simulink model "Q_robot_control_walk_SPT5425"  (R2018b)
settings: Solver=FixedStepAuto  StartTime=0.0  StopTime=10  FixedStep=0.01  RelTol=1e-3
libraries: simulink x3
settings Model: Creator=lsl  LastModifiedBy=lsl

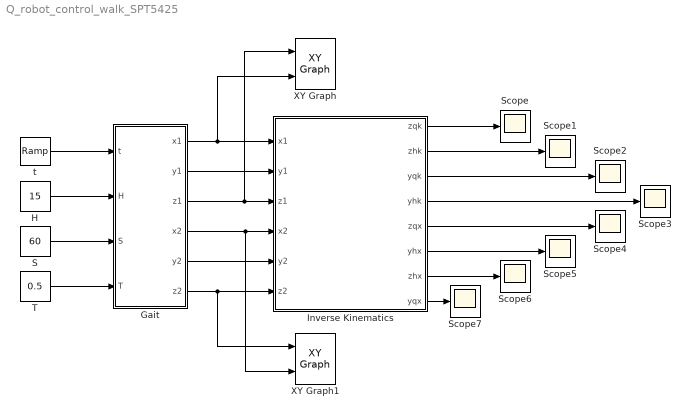
== system Q_robot_control_walk_SPT5425 ==
  Gait : MATLAB Function  TreatAsAtomicUnit=on
  H : Constant  Value=15
  Inverse Kinematics : MATLAB Function  TreatAsAtomicUnit=on
  S : Constant  Value=60
  Scope{,1..7} (8 alike) : Scope
  T : Constant  Value=0.5
  XY Graph : simulink/Sinks/XY Graph  xmin=-100  xmax=100  ymin=-100  ymax=100  st=-1
  XY Graph1 : simulink/Sinks/XY Graph  xmin=-100  xmax=100  ymin=-100  ymax=100  st=-1
  t : simulink/Sources/Ramp  slope=1  start=0  InitialOutput=0
  wires:
  t/1 -> Gait/1(t)
  T/1 -> Gait/4(T)
  Gait/5(y2) -> Inverse Kinematics/5(y2)
  Gait/3(z1) -> XY Graph/1, Inverse Kinematics/3(z1)
  Gait/2(y1) -> Inverse Kinematics/2(y1)
  Gait/1(x1) -> XY Graph/2, Inverse Kinematics/1(x1)
  Inverse Kinematics/6(yhx) -> Scope5/1
  Inverse Kinematics/1(zqk) -> Scope/1
  Inverse Kinematics/7(zhx) -> Scope6/1
  Gait/4(x2) -> XY Graph1/2, Inverse Kinematics/4(x2)
  Gait/6(z2) -> XY Graph1/1, Inverse Kinematics/6(z2)
  Inverse Kinematics/2(zhk) -> Scope1/1
  Inverse Kinematics/3(yqk) -> Scope2/1
  Inverse Kinematics/4(yhk) -> Scope3/1
  Inverse Kinematics/5(zqx) -> Scope4/1
  Inverse Kinematics/8(yqx) -> Scope7/1
  S/1 -> Gait/3(S)
  H/1 -> Gait/2(H)

== matlab function Q_robot_control_walk_SPT5425/Gait ==
  data: t input; H input; x1 output; S input; T input; y1 output; z1 output; x2 output; y2 output; z2 output
function [x1,y1,z1,x2,y2,z2] = Gait_SPT(t,H,S,T)
%x1,y1,z1 摆动相
%x2,y2,z2 支撑相
SwayStatus_Xst=170;
SwayStatus_Yst=43.9;
SwayStatus_Zst=-0.5*S;

SupportingStatus_Xst=170;
SupportingStatus_Yst=43.9;
SupportingStatus_Zst=0.5*S;

if(t>T)
    c=mod(t,T);
else 
    c=t;
end
temp=(t-c)/T;
if(mod(temp,2)==1)
    x1=SwayStatus_Xst-H*(0.5-0.5*cos(2*pi*t/T));
    y1=SwayStatus_Yst;
    if(t>T)
        z1=SwayStatus_Zst+S*(mod(t,T)/T-(sin(2*pi*t/T))/(2*pi));
    else
        z1=SwayStatus_Zst+S*(t/T-(sin(2*pi*t/T))/(2*pi));
    end
    x2=SupportingStatus_Xst;
    y2=SupportingStatus_Yst;
    if(t>T)
        z2=SupportingStatus_Zst-S*mod(t,T)/T;
    else 
       z2=SupportingStatus_Zst-S*t/T;
    end
else 
    x2=SwayStatus_Xst-H*(0.5-0.5*cos(2*pi*t/T));
    y2=SwayStatus_Yst;
    if(t>T)
        z2=SwayStatus_Zst+S*(mod(t,T)/T-(sin(2*pi*t/T))/(2*pi));
    else
        z2=SwayStatus_Zst+S*(t/T-(sin(2*pi*t/T))/(2*pi));
    end
    x1=SupportingStatus_Xst;
    y1=SupportingStatus_Yst;
    if(t>T)
        z1=SupportingStatus_Zst-S*mod(t,T)/T;
    else 
       z1=SupportingStatus_Zst-S*t/T;
    end    
end

== matlab function Q_robot_control_walk_SPT5425/Inverse Kinematics ==
  data: zqk output; x1 input; y1 input; z1 input; x2 input; y2 input; z2 input; zhk output; yqk output; yhk output; zqx output; yhx output; zhx output; yqx output
function [zqk,zhk,yqk,yhk,zqx,yhx,zhx,yqx] = Inverse_Kinematics_SPT(x1,y1,z1,x2,y2,z2)
%x1,y1,z1 摆动相
%x2,y2,z2 支撑相
[~,zqk,zqx]=inverse_kinematics(0,x1,y1,z1);
[~,yhk,yhx]=inverse_kinematics(3,x1,-y1,z1);
[~,zhk,zhx]=inverse_kinematics(2,x2,y2,z2);
[~,yqk,yqx]=inverse_kinematics(1,x2,-y2,z2);   

zqx=-1*zqx;
yhx=-1*yhx;
zhx=-1*zhx;
yqx=-1*yqx;

end

function [theta_1,theta_2,theta_3]=inverse_kinematics(num,x,y,z)
%a1,a2,a3关节长度
a1=43.9;
a2=110;
a3=110;
if(num==1||num==3)
    y=-y;
end
omega=atan2(y,x);
theta_1=asin( -a1/sqrt( power(x,2)+power(y,2) ) )+omega;
theta_3=-acos((power((x*cos(theta_1)+y*sin(theta_1)),2)+power(z,2)-power(a2,2)-power(a3,2))/(2*a2*a3));
fai=atan2(z,(y*sin(theta_1)+x*cos(theta_1)));
theta_2=asin(-a3*sin(theta_3)/sqrt(power((x*cos(theta_1)+y*sin(theta_1)),2)+power(z,2)))-fai;
theta_2=theta_2-pi/4;
theta_3=theta_3+pi/2;

end
